simulink model "zhuansu1000_suddenload_zhw"  (R2015a)
settings: Solver=ode45  StartTime=0.0  StopTime=0.5  RelTol=1e-3
libraries: powerlib x31, powerlib_extras x1
settings Model: Creator=Administrator  LastModifiedBy=Think127
settings DataIOCC: SignalLoggingSaveFormat=ModelDataLogs
settings OptimizationCC: ExpressionDepthLimit=2147483647
settings DebuggingCC: UnderspecifiedInitializationDetection=Classic  MergeDetectMultiDrivingBlocksExec=none  SolverPrmCheckMsg=warning  FcnCallInpInsideContextMsg=UseLocalSettings  StateNameClashWarn=warning
settings GRTTargetCC: CombineOutputUpdateFcns=off  GRTInterface=on

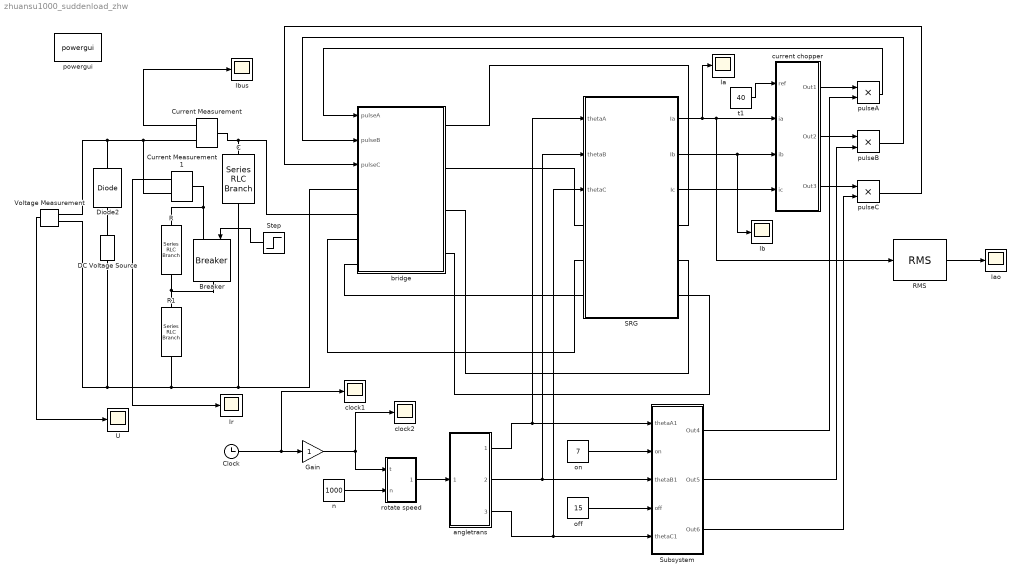
== system zhuansu1000_suddenload_zhw ==
  Breaker : powerlib/Elements/Breaker  InitialState=0  SwitchingTimes="[1/60  5/60]"  External=on  BreakerResistance=0.01  SnubberResistance=1e6  SnubberCapacitance=inf  Measurements=None  MoreParameters=on  NoBreakLoop=off
  "C " : powerlib/Elements/Series RLC Branch  LConnTagsString=__new0  RConnTagsString=__new0  BranchType=C  Resistance=1  Inductance=1.0  SetiL0=off  InitialCurrent=0  Capacitance=1e-3  Setx0=off  InitialVoltage=0  Measurements=None
  Clock : Clock
  Current Measurement : powerlib/Measurements/Current Measurement  PhasorSimulation=off  OutputType=Complex  PSBequivalent=0
  Current Measurement1 : powerlib/Measurements/Current Measurement  PhasorSimulation=off  OutputType=Complex  PSBequivalent=0
  DC Voltage Source : powerlib/Electrical Sources/DC Voltage Source  Amplitude=45  Measurements=None
  Diode2 : powerlib/Power Electronics/Diode  Ron=0.001  Lon=0  Vf=0.8  IC=0  UseSnubber=off  Rs=500  Cs=250e-9  Measurements=off
  Gain : Gain
  Ia : Scope
      settings: YMin=0  YMax=0.6  SaveName=zhuansu1000IA
  Iao : Scope
      settings: YMin=8.47617  YMax=9.36839
  Ib : Scope
      settings: YMin=0  YMax=0.6  SaveName=IA1
  Ibus : Scope
      settings: TimeRange=0.5  YMin=-47500  YMax=2500  SaveName=ScopeData6
  Ir : Scope
      settings: YMin=-6.5  YMax=0.5  SaveName=load_i
  R : powerlib/Elements/Series RLC Branch  LConnTagsString=__new0  RConnTagsString=__new0  BranchType=R  Resistance=50  Inductance=1.0  SetiL0=off  InitialCurrent=0  Capacitance=1.0  Setx0=off  InitialVoltage=0  Measurements=None
  R1 : powerlib/Elements/Series RLC Branch  LConnTagsString=__new0  RConnTagsString=__new0  BranchType=R  Resistance=50  Inductance=1.0  SetiL0=off  InitialCurrent=0  Capacitance=1.0  Setx0=off  InitialVoltage=0  Measurements=None
  RMS : powerlib_extras/Measurements/RMS  f1=5
  SRG : Subsystem
  Step : Step  Time=0.25  SampleTime=0
  Subsystem : Subsystem
  U : Scope
      settings: YMin=-25  YMax=350  SaveName=zhuansu1000U
  Voltage Measurement : powerlib/Measurements/Voltage Measurement  PhasorSimulation=off  OutputType=Complex  PSBequivalent=0
  angletrans : Subsystem
  bridge : Subsystem
  clock1 : Scope
      settings: YMin=0.00565  YMax=0.0064  SaveName=ScopeData2
  clock2 : Scope
      settings: YMin=0.001  YMax=0.00215  SaveName=ScopeData3
  current chopper : Subsystem
  n : Constant  Value=1000
  off : Constant  Value=15
  on : Constant  Value=7
  powergui : powerlib/powergui  Priority=1  SimulationMode=Continuous  SolverType=Tustin/Backward Euler (TBE)  SampleTime=50e-6  frequency=60  SPID=off  DisableSnubberDevices=off  DisableRonSwitches=off  DisableVfSwitches=off  SwTol=0  DisplayEquations=off  Interpol=off  methode=off  Ts=0  FunctionMessages=off  echomessages=off  HookPort=off  EnableUseOfTLC=off  x0status=blocks  frequencyindice=0  Pbase=100e6  ErrMax=1e-4  Iterations=50  UnitsV=kV  UnitsW=MW  buscounter=0  RestoreLinks=warning  ResistiveCurrentMeasurement=off  Frange=[0:2:500]  Ylog=off  Xlog=on  ShowGrid=off  save=off  variable=ZData  structure=0  ZoomFFT=on  StartTime=0.0  cycles=1  DisplayStyle=1  fundamental=60  FreqAxis=off  MaxFrequency=1000  frequencyindicesteady=1  RmsSteady=1  display=off
  pulseA : Product  RndMeth=Zero
  pulseB : Product  RndMeth=Zero
  pulseC : Product  RndMeth=Zero
  rotate speed : Subsystem
  t1 : Constant  Value=40
  wires:
  SRG/1(Ia) -> current chopper/2(ia), RMS/1, Ia/1
  SRG/2(Ib) -> current chopper/3(ib), Ib/1
  SRG/3(Ic) -> current chopper/4(ic)
  rotate speed/1(theta) -> angletrans/1(theta)
  n/1 -> rotate speed/2(n)
  on/1 -> Subsystem/2(on)
  off/1 -> Subsystem/4(off)
  angletrans/1(thetaA) -> Subsystem/1(thetaA1), SRG/1(thetaA)
  angletrans/2(thetaB) -> Subsystem/3(thetaB1), SRG/2(thetaB)
  angletrans/3(thetaC) -> Subsystem/5(thetaC1), SRG/3(thetaC)
  Voltage Measurement/1 -> U/1
  Subsystem/1(Out4) -> pulseA/2
  Subsystem/3(Out6) -> pulseC/2
  Subsystem/2(Out5) -> pulseB/2
  current chopper/1(Out1) -> pulseA/1
  current chopper/2(Out2) -> pulseB/1
  current chopper/3(Out3) -> pulseC/1
  pulseB/1 -> bridge/2(pulseB)
  pulseC/1 -> bridge/3(pulseC)
  pulseA/1 -> bridge/1(pulseA)
  t1/1 -> current chopper/1(ref)
  Gain/1 -> rotate speed/1(t), clock2/1
  Clock/1 -> Gain/1, clock1/1
  RMS/1 -> Iao/1
  Current Measurement/1 -> Ibus/1
  Current Measurement1/1 -> Ir/1
  Step/1 -> Breaker/1
  connections:
  Diode2/LConn1 -- DC Voltage Source/RConn1
  "C "/LConn1 -- bridge/LConn2 -- Current Measurement/LConn1
  bridge/RConn2 -- SRG/LConn1
  bridge/RConn1 -- SRG/RConn1
  bridge/LConn3 -- SRG/LConn2
  bridge/LConn4 -- SRG/LConn3
  bridge/RConn4 -- SRG/RConn3
  bridge/RConn3 -- SRG/RConn2
  bridge/LConn1 -- "C "/RConn1 -- R1/RConn1 -- DC Voltage Source/LConn1 -- Voltage Measurement/LConn2
  Current Measurement/RConn1 -- Diode2/RConn1 -- Voltage Measurement/LConn1 -- Current Measurement1/RConn1
  Current Measurement1/LConn1 -- R/LConn1 -- Breaker/LConn1
  R1/LConn1 -- Breaker/RConn1 -- R/RConn1

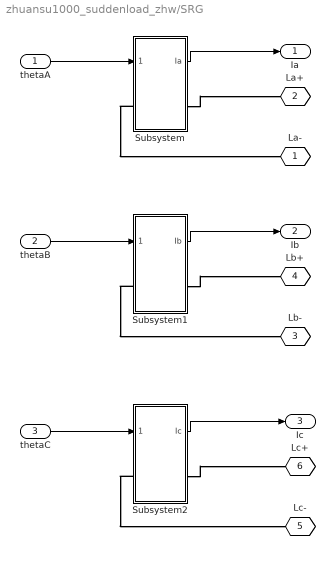
== system zhuansu1000_suddenload_zhw/SRG ==
  thetaA : Inport
  thetaB : Inport  Port=2
  thetaC : Inport  Port=3
  Subsystem : Subsystem
  Subsystem1 : Subsystem
  Subsystem2 : Subsystem
  La- : PMIOPort  Tag=PMCPort  Port=1  Side=Left
  La+ : PMIOPort  Tag=PMCPort  Port=2  Side=Right
  Lb- : PMIOPort  Tag=PMCPort  Port=3  Side=Left
  Lb+ : PMIOPort  Tag=PMCPort  Port=4  Side=Right
  Lc- : PMIOPort  Tag=PMCPort  Port=5  Side=Left
  Lc+ : PMIOPort  Tag=PMCPort  Port=6  Side=Right
  Ia : Outport
  Ib : Outport  Port=2
  Ic : Outport  Port=3
  wires:
  thetaA/1 -> Subsystem/1(thetaA)
  Subsystem/1(Ia) -> Ia/1
  thetaB/1 -> Subsystem1/1(thetaB)
  Subsystem1/1(Ib) -> Ib/1
  thetaC/1 -> Subsystem2/1(thetaC)
  Subsystem2/1(Ic) -> Ic/1
  connections:
  Subsystem/LConn1 -- La-/RConn1
  Subsystem/RConn1 -- La+/RConn1
  Subsystem1/LConn1 -- Lb-/RConn1
  Subsystem1/RConn1 -- Lb+/RConn1
  Subsystem2/LConn1 -- Lc-/RConn1
  Subsystem2/RConn1 -- Lc+/RConn1

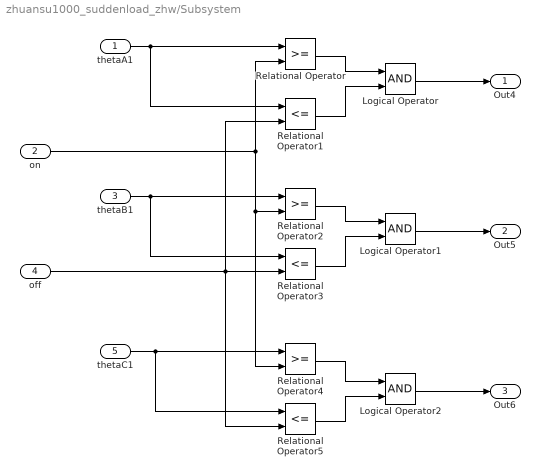
== system zhuansu1000_suddenload_zhw/Subsystem ==
  thetaA1 : Inport
  on : Inport  Port=2
  thetaB1 : Inport  Port=3
  off : Inport  Port=4
  thetaC1 : Inport  Port=5
  Logical Operator : Logic  AllPortsSameDT=off  OutDataTypeStr=boolean
  Logical Operator1 : Logic  AllPortsSameDT=off  OutDataTypeStr=boolean
  Logical Operator2 : Logic  AllPortsSameDT=off  OutDataTypeStr=boolean
  Relational Operator : RelationalOperator  OutDataTypeStr=boolean
  Relational Operator1 : RelationalOperator  Operator=<=  OutDataTypeStr=boolean
  Relational Operator2 : RelationalOperator  OutDataTypeStr=boolean
  Relational Operator3 : RelationalOperator  Operator=<=  OutDataTypeStr=boolean
  Relational Operator4 : RelationalOperator  OutDataTypeStr=boolean
  Relational Operator5 : RelationalOperator  Operator=<=  OutDataTypeStr=boolean
  Out4 : Outport
  Out5 : Outport  Port=2
  Out6 : Outport  Port=3
  wires:
  thetaA1/1 -> Relational Operator/1, Relational Operator1/1
  thetaB1/1 -> Relational Operator2/1, Relational Operator3/1
  thetaC1/1 -> Relational Operator4/1, Relational Operator5/1
  on/1 -> Relational Operator/2, Relational Operator2/2, Relational Operator4/2
  off/1 -> Relational Operator1/2, Relational Operator3/2, Relational Operator5/2
  Relational Operator/1 -> Logical Operator/1
  Relational Operator1/1 -> Logical Operator/2
  Relational Operator2/1 -> Logical Operator1/1
  Relational Operator3/1 -> Logical Operator1/2
  Relational Operator4/1 -> Logical Operator2/1
  Relational Operator5/1 -> Logical Operator2/2
  Logical Operator/1 -> Out4/1
  Logical Operator1/1 -> Out5/1
  Logical Operator2/1 -> Out6/1

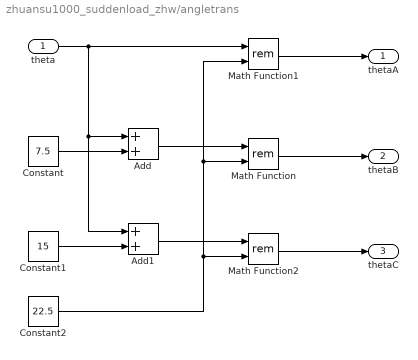
== system zhuansu1000_suddenload_zhw/angletrans ==
  theta : Inport
  Add : Sum
  Add1 : Sum
  Constant : Constant  Value=7.5
  Constant1 : Constant  Value=15
  Constant2 : Constant  Value=22.5
  Math Function : Math  Operator=rem  SaturateOnIntegerOverflow=on
  Math Function1 : Math  Operator=rem  SaturateOnIntegerOverflow=on
  Math Function2 : Math  Operator=rem  SaturateOnIntegerOverflow=on
  thetaA : Outport
  thetaB : Outport  Port=2
  thetaC : Outport  Port=3
  wires:
  Add1/1 -> Math Function2/1
  Add/1 -> Math Function/1
  theta/1 -> Math Function1/1, Add1/1, Add/1
  Constant/1 -> Add/2
  Constant1/1 -> Add1/2
  Constant2/1 -> Math Function2/2, Math Function/2, Math Function1/2
  Math Function2/1 -> thetaC/1
  Math Function/1 -> thetaB/1
  Math Function1/1 -> thetaA/1

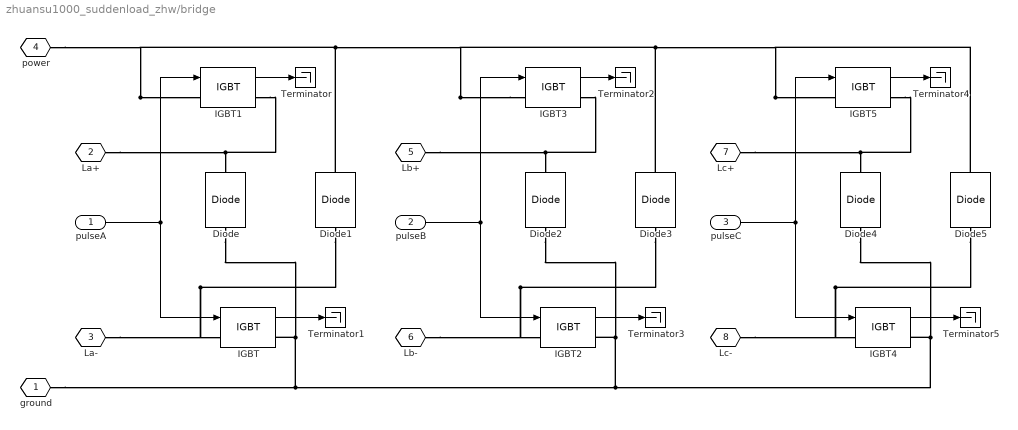
== system zhuansu1000_suddenload_zhw/bridge ==
  pulseA : Inport
  pulseB : Inport  Port=2
  pulseC : Inport  Port=3
  Diode{,1..5} (6 alike) : powerlib/Power Electronics/Diode  Ron=0.001  Lon=0  Vf=0.8  IC=0  UseSnubber=off  Rs=500  Cs=250e-9  Measurements=off
  IGBT{,1..5} (6 alike) : powerlib/Power Electronics/IGBT  Ron=0.001  Lon=0  Vf=1  Tf=1e-6  Tt=2e-6  IC=0  Rs=1e5  Cs=inf  Measurements=on
  Terminator{,1..5} (6 alike) : Terminator
  ground : PMIOPort  Tag=PMCPort  Port=1  Side=Left
  La+ : PMIOPort  Tag=PMCPort  Port=2  Side=Right
  La- : PMIOPort  Tag=PMCPort  Port=3  Side=Right
  power : PMIOPort  Tag=PMCPort  Port=4  Side=Left
  Lb+ : PMIOPort  Tag=PMCPort  Port=5  Side=Right
  Lb- : PMIOPort  Tag=PMCPort  Port=6  Side=Left
  Lc+ : PMIOPort  Tag=PMCPort  Port=7  Side=Right
  Lc- : PMIOPort  Tag=PMCPort  Port=8  Side=Left
  wires:
  IGBT4/1 -> Terminator5/1
  IGBT5/1 -> Terminator4/1
  pulseC/1 -> IGBT4/1, IGBT5/1
  IGBT2/1 -> Terminator3/1
  IGBT3/1 -> Terminator2/1
  pulseB/1 -> IGBT2/1, IGBT3/1
  IGBT/1 -> Terminator1/1
  IGBT1/1 -> Terminator/1
  pulseA/1 -> IGBT/1, IGBT1/1
  connections:
  Lc-/RConn1 -- IGBT4/LConn1 -- Diode5/LConn1
  Lc+/RConn1 -- IGBT5/RConn1 -- Diode4/RConn1
  Lb-/RConn1 -- IGBT2/LConn1 -- Diode3/LConn1
  IGBT3/RConn1 -- Lb+/RConn1 -- Diode2/RConn1
  IGBT3/LConn1 -- Diode5/RConn1 -- IGBT5/LConn1 -- Diode3/RConn1 -- Diode1/RConn1 -- IGBT1/LConn1 -- power/RConn1
  La-/RConn1 -- IGBT/LConn1 -- Diode1/LConn1
  La+/RConn1 -- IGBT1/RConn1 -- Diode/RConn1
  IGBT2/RConn1 -- Diode2/LConn1 -- IGBT/RConn1 -- Diode/LConn1 -- ground/RConn1 -- IGBT4/RConn1 -- Diode4/LConn1

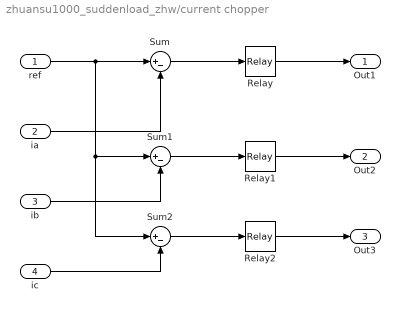
== system zhuansu1000_suddenload_zhw/current chopper ==
  ref : Inport
  ia : Inport  Port=2
  ib : Inport  Port=3
  ic : Inport  Port=4
  Relay : Relay  OnSwitchValue=2  OffSwitchValue=-2
  Relay1 : Relay  OnSwitchValue=2  OffSwitchValue=-2
  Relay2 : Relay  OnSwitchValue=2  OffSwitchValue=-2
  Sum : Sum  Inputs=|+-
  Sum1 : Sum  Inputs=|+-
  Sum2 : Sum  Inputs=|+-
  Out1 : Outport
  Out2 : Outport  Port=2
  Out3 : Outport  Port=3
  wires:
  Relay/1 -> Out1/1
  Relay1/1 -> Out2/1
  Relay2/1 -> Out3/1
  Sum/1 -> Relay/1
  Sum1/1 -> Relay1/1
  Sum2/1 -> Relay2/1
  ref/1 -> Sum/1, Sum2/1, Sum1/1
  ia/1 -> Sum/2
  ib/1 -> Sum1/2
  ic/1 -> Sum2/2

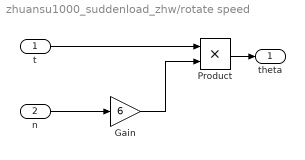
== system zhuansu1000_suddenload_zhw/rotate speed ==
  t : Inport
  n : Inport  Port=2
  Gain : Gain  Gain=6
  Product : Product  RndMeth=Zero
  theta : Outport
  wires:
  n/1 -> Gain/1
  Gain/1 -> Product/2
  t/1 -> Product/1
  Product/1 -> theta/1

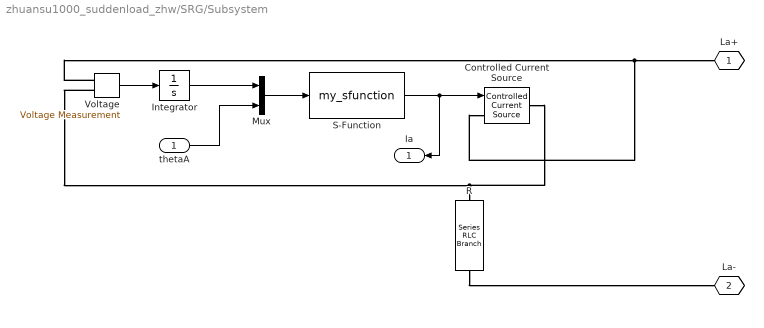
== system zhuansu1000_suddenload_zhw/SRG/Subsystem ==
  thetaA : Inport
  Controlled Current Source : powerlib/Electrical Sources/Controlled Current Source  Initialize=on  Source_Type=AC  Amplitude=0  Phase=0  Frequency=0  Measurements=None
  Integrator : Integrator  LimitOutput=on  LowerSaturationLimit=0
  Mux : Mux  Inputs=2
  R : powerlib/Elements/Series RLC Branch  LConnTagsString=__new0  RConnTagsString=__new0  BranchType=R  Resistance=0.0261014  Inductance=1.0  SetiL0=off  InitialCurrent=0  Capacitance=1.0  Setx0=off  InitialVoltage=0  Measurements=None
  S-Function : S-Function  FunctionName=my_sfunction
  Voltage : powerlib/Measurements/Voltage Measurement  PhasorSimulation=off  OutputType=Complex  PSBequivalent=0
  La+ : PMIOPort  Tag=PMCPort  Port=1  Side=Right
  La- : PMIOPort  Tag=PMCPort  Port=2  Side=Left
  Ia : Outport
  wires:
  Mux/1 -> S-Function/1
  Integrator/1 -> Mux/1
  thetaA/1 -> Mux/2
  S-Function/1 -> Ia/1, Controlled Current Source/1
  Voltage/1 -> Integrator/1
  connections:
  R/LConn1 -- Controlled Current Source/RConn1 -- Voltage/LConn2
  Voltage/LConn1 -- La+/RConn1 -- Controlled Current Source/LConn1
  R/RConn1 -- La-/RConn1

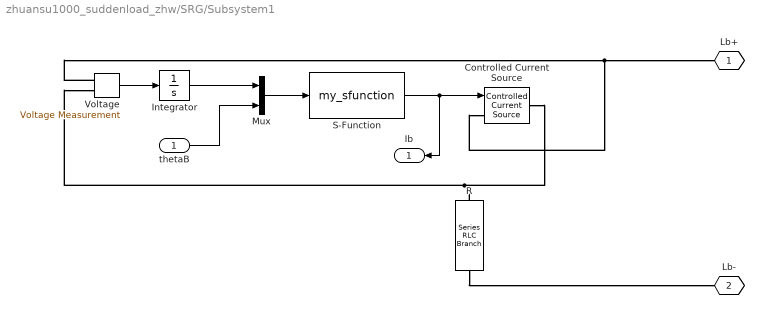
== system zhuansu1000_suddenload_zhw/SRG/Subsystem1 ==
  thetaB : Inport
  Controlled Current Source : powerlib/Electrical Sources/Controlled Current Source  Initialize=on  Source_Type=AC  Amplitude=0  Phase=0  Frequency=0  Measurements=None
  Integrator : Integrator  LimitOutput=on  LowerSaturationLimit=0
  Mux : Mux  Inputs=2
  R : powerlib/Elements/Series RLC Branch  LConnTagsString=__new0  RConnTagsString=__new0  BranchType=R  Resistance=0.0261014  Inductance=1.0  SetiL0=off  InitialCurrent=0  Capacitance=1.0  Setx0=off  InitialVoltage=0  Measurements=None
  S-Function : S-Function  FunctionName=my_sfunction
  Voltage : powerlib/Measurements/Voltage Measurement  PhasorSimulation=off  OutputType=Complex  PSBequivalent=0
  Lb+ : PMIOPort  Tag=PMCPort  Port=1  Side=Right
  Lb- : PMIOPort  Tag=PMCPort  Port=2  Side=Left
  Ib : Outport
  wires:
  Mux/1 -> S-Function/1
  Integrator/1 -> Mux/1
  thetaB/1 -> Mux/2
  S-Function/1 -> Ib/1, Controlled Current Source/1
  Voltage/1 -> Integrator/1
  connections:
  R/LConn1 -- Voltage/LConn2 -- Controlled Current Source/RConn1
  Voltage/LConn1 -- Lb+/RConn1 -- Controlled Current Source/LConn1
  R/RConn1 -- Lb-/RConn1

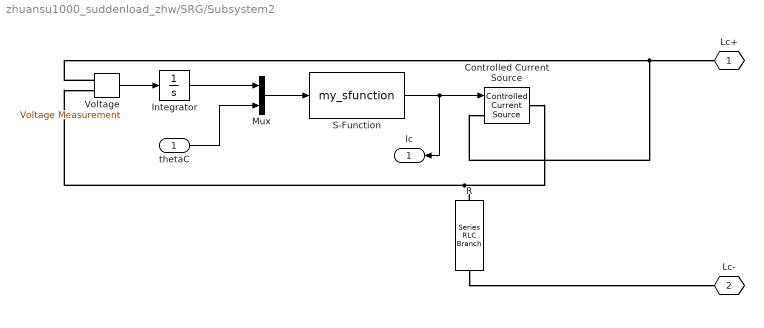
== system zhuansu1000_suddenload_zhw/SRG/Subsystem2 ==
  thetaC : Inport
  Controlled Current Source : powerlib/Electrical Sources/Controlled Current Source  Initialize=on  Source_Type=AC  Amplitude=0  Phase=0  Frequency=0  Measurements=None
  Integrator : Integrator  LimitOutput=on  LowerSaturationLimit=0
  Mux : Mux  Inputs=2
  R : powerlib/Elements/Series RLC Branch  LConnTagsString=__new0  RConnTagsString=__new0  BranchType=R  Resistance=0.0261014  Inductance=1.0  SetiL0=off  InitialCurrent=0  Capacitance=1.0  Setx0=off  InitialVoltage=0  Measurements=None
  S-Function : S-Function  FunctionName=my_sfunction
  Voltage : powerlib/Measurements/Voltage Measurement  PhasorSimulation=off  OutputType=Complex  PSBequivalent=0
  Lc+ : PMIOPort  Tag=PMCPort  Port=1  Side=Right
  Lc- : PMIOPort  Tag=PMCPort  Port=2  Side=Left
  Ic : Outport
  wires:
  Mux/1 -> S-Function/1
  Integrator/1 -> Mux/1
  thetaC/1 -> Mux/2
  S-Function/1 -> Ic/1, Controlled Current Source/1
  Voltage/1 -> Integrator/1
  connections:
  R/LConn1 -- Voltage/LConn2 -- Controlled Current Source/RConn1
  Voltage/LConn1 -- Lc+/RConn1 -- Controlled Current Source/LConn1
  R/RConn1 -- Lc-/RConn1
